simulink model "lab11sim"  (R2020a)
settings: Solver=VariableStepAuto  StartTime=0.0  StopTime=30  RelTol=1e-3
settings Model: Creator=ariana  LastModifiedBy=ariana

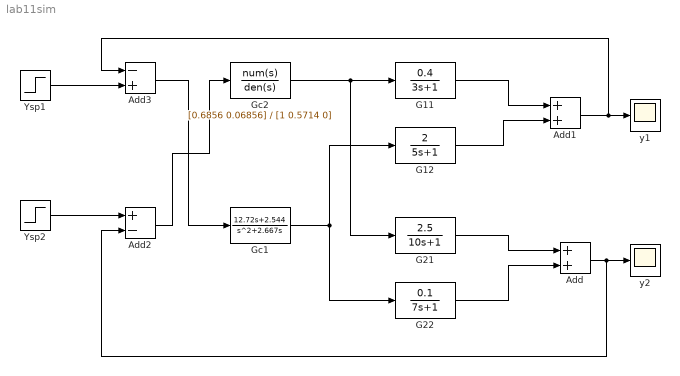
== system lab11sim ==
  " G12" : TransferFcn  Numerator=[2]  Denominator=[5 1]
  " G21" : TransferFcn  Numerator=[2.5]  Denominator=[10 1]
  " G22" : TransferFcn  Numerator=[0.1]  Denominator=[7 1]
  " Gc1" : TransferFcn  Numerator=[12.72 2.544]  Denominator=[1 2.667 0]
  Add : Sum
  Add1 : Sum
  Add2 : Sum  Inputs=+-
  Add3 : Sum  Inputs=-+
  G11 : TransferFcn  Numerator=[0.4]  Denominator=[3 1]
  "Gc2 " : TransferFcn  Numerator=[0.6856 0.06856]  Denominator=[1 0.5714 0]
  Ysp1 : Step  Time=0  SampleTime=0
  Ysp2 : Step  Time=0  SampleTime=0
  y1 : Scope
  y2 : Scope
  wires:
  Ysp1/1 -> Add3/2
  Ysp2/1 -> Add2/1
  Add/1 -> Add2/2, y2/1
  Add1/1 -> Add3/1, y1/1
  G11/1 -> Add1/1
  " G12"/1 -> Add1/2
  " G21"/1 -> Add/1
  " G22"/1 -> Add/2
  "Gc2 "/1 -> " G21"/1, G11/1
  " Gc1"/1 -> " G22"/1, " G12"/1
  Add3/1 -> " Gc1"/1
  Add2/1 -> "Gc2 "/1
